simulink model "Project_parameter_Estimation_motor_model"  (R2023b)
settings: Solver=VariableStepAuto  StartTime=0.0  StopTime=25  MaxStep=0.001  RelTol=1e-3
undefined symbols (not defined in the file or in its folder): De, Je, Kb, Kt, La, Ra
libraries: SignalEditorBlockLib x1
settings Model: Creator=AHMED MOHSEN  LastModifiedBy=AHMED MOHSEN

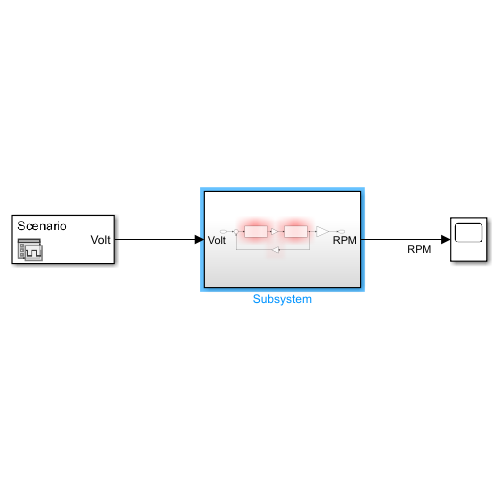
[thumbnail: Simulink's stored preview of the top-level diagram]
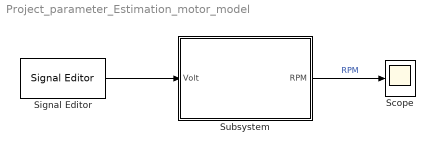
== system Project_parameter_Estimation_motor_model ==
  Scope : Scope
  Signal Editor : SignalEditorBlockLib/Signal Editor  FileName=volt_signal_parameter_estimation.mat  ActiveScenario=Scenario  ActiveSignal=Volt  IsBus=off  OutputBusObjectStr=Bus: BusObject  SampleTime=0  Interpolate=off  ZeroCross=off  OutputAfterFinalValue=Setting to zero  Unit=inherit  PreserveSignalName=on  ApplySigPropsToAllScenarios=on  ApplySigPropsToAllSignals=off
  Subsystem : Subsystem
  wires:
  Signal Editor/1 -> Subsystem/1(Volt)
  Subsystem/1(RPM) -> Scope/1  "RPM"

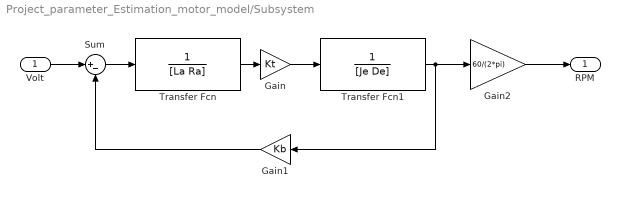
== system Project_parameter_Estimation_motor_model/Subsystem ==
  Volt : Inport
  Gain : Gain  Gain=Kt
  Gain1 : Gain  Gain=Kb
  Gain2 : Gain  Gain=60/(2*pi)
  Sum : Sum  Inputs=|+-
  Transfer Fcn : TransferFcn  Denominator=[La Ra]
  Transfer Fcn1 : TransferFcn  Denominator=[Je De]
  RPM : Outport
  wires:
  Transfer Fcn/1 -> Gain/1
  Sum/1 -> Transfer Fcn/1
  Volt/1 -> Sum/1
  Gain1/1 -> Sum/2
  Transfer Fcn1/1 -> Gain2/1, Gain1/1
  Gain/1 -> Transfer Fcn1/1
  Gain2/1 -> RPM/1
